simulink model "b2_df2sos_mdl"  (R2020a)
settings: Solver=VariableStepAuto  StartTime=0.0  StopTime=10.0  RelTol=1e-3
settings Model: Creator=soymarwin  LastModifiedBy=soymarwin

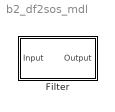
== system b2_df2sos_mdl ==
  Filter : Subsystem  Tag=FilterWizardSubSystem

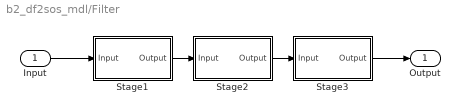
== system b2_df2sos_mdl/Filter ==
  Input : Inport
  Stage1 : Subsystem  Tag=FilterWizardSubSystem
      settings: ErrorFcn=dspFilterRealizedInBasicElemsAlgLoopErrFcnCallback
  Stage2 : Subsystem  Tag=FilterWizardSubSystem
      settings: ErrorFcn=dspFilterRealizedInBasicElemsAlgLoopErrFcnCallback
  Stage3 : Subsystem  Tag=FilterWizardSubSystem
      settings: ErrorFcn=dspFilterRealizedInBasicElemsAlgLoopErrFcnCallback
  Output : Outport
  wires:
  Input/1 -> Stage1/1(Input)
  Stage1/1(Output) -> Stage2/1(Input)
  Stage2/1(Output) -> Stage3/1(Input)
  Stage3/1(Output) -> Output/1

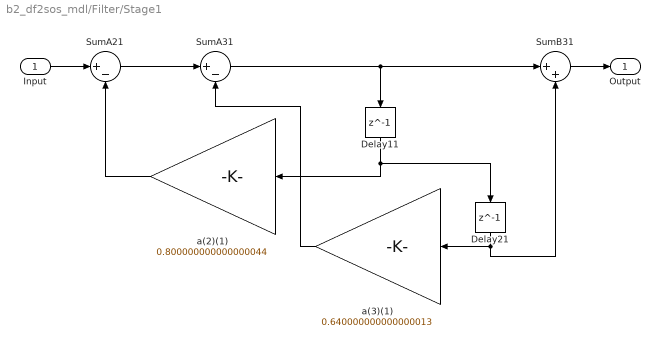
== system b2_df2sos_mdl/Filter/Stage1 ==
  Input : Inport
  Delay11 : Delay  DelayLength=1  InitialCondition=0
  Delay21 : Delay  DelayLength=1  InitialCondition=0
  SumA21 : Sum  Inputs=|+-  RndMeth=Nearest  SaturateOnIntegerOverflow=on  OutDataTypeStr=Inherit: Same as first input
  SumA31 : Sum  Inputs=|+-  RndMeth=Nearest  SaturateOnIntegerOverflow=on  OutDataTypeStr=Inherit: Same as first input
  SumB31 : Sum  Inputs=|++  RndMeth=Nearest  SaturateOnIntegerOverflow=on  OutDataTypeStr=Inherit: Same as first input
  a(2)(1) : Gain  Gain=0.800000000000000044  ParamDataTypeStr=double  RndMeth=Nearest  SaturateOnIntegerOverflow=on  OutDataTypeStr=Inherit: Same as input
  a(3)(1) : Gain  Gain=0.640000000000000013  ParamDataTypeStr=double  RndMeth=Nearest  SaturateOnIntegerOverflow=on  OutDataTypeStr=Inherit: Same as input
  Output : Outport
  wires:
  SumA21/1 -> SumA31/1
  Input/1 -> SumA21/1
  SumB31/1 -> Output/1
  a(2)(1)/1 -> SumA21/2
  a(3)(1)/1 -> SumA31/2
  SumA31/1 -> Delay11/1, SumB31/1
  Delay11/1 -> Delay21/1, a(2)(1)/1
  Delay21/1 -> SumB31/2, a(3)(1)/1

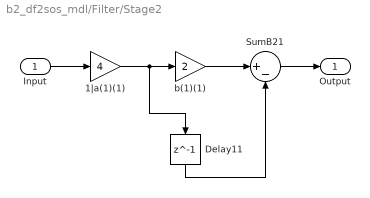
== system b2_df2sos_mdl/Filter/Stage2 ==
  Input : Inport
  1|a(1)(1) : Gain  Gain=4  ParamDataTypeStr=double  RndMeth=Nearest  SaturateOnIntegerOverflow=on  OutDataTypeStr=Inherit: Same as input
  Delay11 : Delay  DelayLength=1  InitialCondition=0
  SumB21 : Sum  Inputs=|+-  RndMeth=Nearest  SaturateOnIntegerOverflow=on  OutDataTypeStr=Inherit: Same as first input
  b(1)(1) : Gain  Gain=2  ParamDataTypeStr=double  RndMeth=Nearest  SaturateOnIntegerOverflow=on  OutDataTypeStr=Inherit: Same as input
  Output : Outport
  wires:
  Input/1 -> 1|a(1)(1)/1
  b(1)(1)/1 -> SumB21/1
  SumB21/1 -> Output/1
  Delay11/1 -> SumB21/2
  1|a(1)(1)/1 -> Delay11/1, b(1)(1)/1

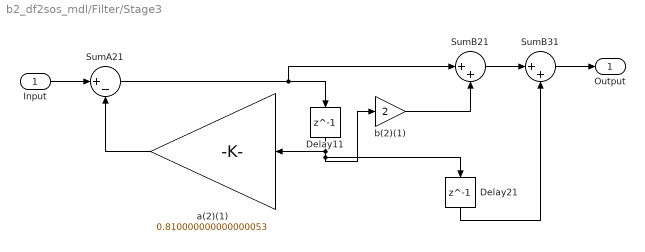
== system b2_df2sos_mdl/Filter/Stage3 ==
  Input : Inport
  Delay11 : Delay  DelayLength=1  InitialCondition=0
  Delay21 : Delay  DelayLength=1  InitialCondition=0
  SumA21 : Sum  Inputs=|+-  RndMeth=Nearest  SaturateOnIntegerOverflow=on  OutDataTypeStr=Inherit: Same as first input
  SumB21 : Sum  Inputs=|++  RndMeth=Nearest  SaturateOnIntegerOverflow=on  OutDataTypeStr=Inherit: Same as first input
  SumB31 : Sum  Inputs=|++  RndMeth=Nearest  SaturateOnIntegerOverflow=on  OutDataTypeStr=Inherit: Same as first input
  a(2)(1) : Gain  Gain=0.810000000000000053  ParamDataTypeStr=double  RndMeth=Nearest  SaturateOnIntegerOverflow=on  OutDataTypeStr=Inherit: Same as input
  b(2)(1) : Gain  Gain=2  ParamDataTypeStr=double  RndMeth=Nearest  SaturateOnIntegerOverflow=on  OutDataTypeStr=Inherit: Same as input
  Output : Outport
  wires:
  a(2)(1)/1 -> SumA21/2
  Delay21/1 -> SumB31/2
  b(2)(1)/1 -> SumB21/2
  SumB31/1 -> Output/1
  SumB21/1 -> SumB31/1
  SumA21/1 -> SumB21/1, Delay11/1
  Delay11/1 -> b(2)(1)/1, Delay21/1, a(2)(1)/1
  Input/1 -> SumA21/1
